simulink model "PR"  (R2025b)
settings: Solver=ode45  StartTime=0.0  StopTime=10.0  MaxStep=1e-3  RelTol=1e-3
values from neighbouring files (symbols this model uses):
  Fc = 0    [PR.m]    (also in PR1.m = 0.2)
settings Model: Creator=juani  LastModifiedBy=juani

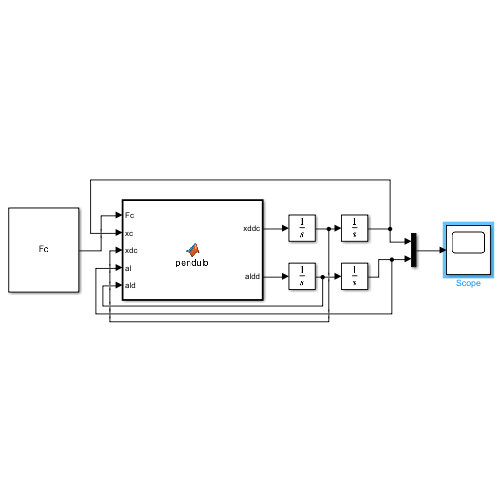
[thumbnail: Simulink's stored preview of the top-level diagram]
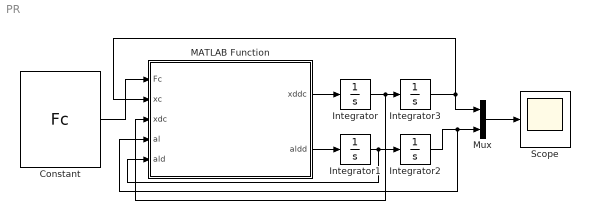
== system PR ==
  Constant : Constant  Value=Fc
  Integrator : Integrator
  Integrator1 : Integrator
  Integrator2 : Integrator  InitialCondition=0.01745
  Integrator3 : Integrator
  MATLAB Function : MATLAB Function  TreatAsAtomicUnit=on
  Mux : Mux  Inputs=2
  Scope : Scope
      settings: ActiveDisplayYMinimum=-12.449694099466882  ActiveDisplayYMaximum=112.04724689520197
  wires:
  MATLAB Function/1(xddc) -> Integrator/1
  MATLAB Function/2(aldd) -> Integrator1/1
  Integrator1/1 -> Integrator2/1, MATLAB Function/5(ald)
  Constant/1 -> MATLAB Function/1(Fc)
  Integrator/1 -> MATLAB Function/3(xdc), Integrator3/1
  Integrator2/1 -> MATLAB Function/4(al), Mux/2
  Integrator3/1 -> Mux/1, MATLAB Function/2(xc)
  Mux/1 -> Scope/1

== matlab function PR/MATLAB Function ==
  data: Fc input; xddc output; xc input; xdc input; al input; ald input; aldd output
function[xddc, aldd]=pendulo(Fc,xc,xdc,al,ald)

% Parámetros
Ip=0.0079;
Mc=0.7031;
lp=0.3302;
Mp=0.23;
Beq=4.3;
g=9.81;
Bp=0.0024;

% Denominador 
d=(Mc+Mp)*Ip+Mc*Mp*lp^2+Mp^2*lp^2*sin(al)^2;

% Derivada y operaciones de x
x=(Ip + Mp*lp^2)*Fc ...
     + Mp^2*lp^2*g*cos(al)*sin(al) ...
     - (Ip + Mp*lp^2)*Beq*xdc ...
     - (Ip*Mp*lp - Mp^2*lp^3)*ald^2*sin(al) ...
     - Mp*lp*ald*cos(al)*Bp;
xddc=x/d;

% Derivada y operaciones de alpha
a=(Mc + Mp)*Mp*g*lp*sin(al) ...
     - (Mc + Mp)*Bp*ald ...
     + Fc*Mp*lp*cos(al) ...
     - Mp^2*lp^2*ald^2*sin(al)*cos(al) ...
     - Beq*Mp*lp*xdc*cos(al);
aldd=a/d;
end
